simulink model "Tire_model_pacejka"  (R2020b)
settings: Solver=VariableStepAuto  StartTime=0.0  StopTime=10.0  RelTol=1e-3
InitFcn:
  | vals_struct = load('lateral_coeff_lut.mat');
  | sa_x = vals_struct.sa_x;
  | load_y = vals_struct.load_y;
  | load_y = flip(load_y);
  | lateral_coeff = vals_struct.lat_coeff;
  | lateral_coeff = fliplr(lateral_coeff);
  | vals_struct = load('aligning_torque_lut.mat');
  | aligning_torque = vals_struct.aligning_torque;
  | aligning_torque = fliplr(aligning_torque);
settings Model: Creator=yafta  LastModifiedBy=Matthew

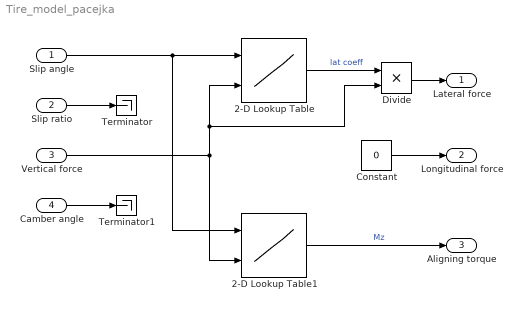
== system Tire_model_pacejka ==
  Slip angle : Inport
  Slip ratio : Inport  Port=2
  Vertical force : Inport  Port=3
  Camber angle : Inport  Port=4
  2-D Lookup Table : Lookup_n-D  BreakpointsForDimension1=sa_x  BreakpointsForDimension2=load_y  Table=lateral_coeff  InternalRulePriority=Speed  RndMeth=Simplest  InputSameDT=on
      settings: InputPortMap=u0,u1
  2-D Lookup Table1 : Lookup_n-D  BreakpointsForDimension1=sa_x  BreakpointsForDimension2=load_y  Table=aligning_torque  InternalRulePriority=Speed  RndMeth=Simplest  InputSameDT=on
      settings: InputPortMap=u0,u1
  Constant : Constant  Value=0
  Divide : Product  Inputs=**
  Terminator : Terminator
  Terminator1 : Terminator
  Lateral force : Outport
  Longitudinal force : Outport  Port=2
  Aligning torque : Outport  Port=3
  wires:
  Constant/1 -> Longitudinal force/1
  Slip ratio/1 -> Terminator/1
  Camber angle/1 -> Terminator1/1
  Vertical force/1 -> Divide/2, 2-D Lookup Table/2, 2-D Lookup Table1/2
  Slip angle/1 -> 2-D Lookup Table1/1, 2-D Lookup Table/1
  2-D Lookup Table1/1 -> Aligning torque/1  "Mz"
  2-D Lookup Table/1 -> Divide/1  "lat coeff"
  Divide/1 -> Lateral force/1
